simulink model "px4demo_attitude_plant"  (R2017b)
settings: Solver=ode3  StartTime=0.0  StopTime=20  RelTol=1e-3  EnableMultiTasking=on
libraries: aerolibobsolete x1, aerolibatmos2 x1, aerolibnav x1
Description:
  | PX4 PSP Example Model for a Attitude Control/Plant Model
  | 
  | ATTITUDE CONTROL PLANT Top-Level System
settings Model: Creator=skuznick  LastModifiedBy=skuznick
settings DataIOCC: LimitDataPoints=on  SaveFormat=Array
settings OptimizationCC: LifeSpan=1.0
settings DebuggingCC: SolverPrmCheckMsg=warning  AllowSymbolicDim=off  SFUnexpectedBacktrackingDiag=warning  SFNoUnconditionalDefaultTransitionDiag=warning  SFExecutionAtInitializationDiag=none
settings HardwareCC: ProdBitPerPointer=32  ProdBitPerSizeT=32  ProdBitPerPtrDiffT=32  ProdLargestAtomicInteger=Long  ProdLargestAtomicFloat=Double  ProdIntDivRoundTo=Undefined  ProdWordSize=32  ProdHWDeviceType=ARM Compatible->ARM Cortex
settings ModelReferenceCC: PropagateSignalLabelsOutOfModel=off
settings CodeAppCC: StateflowObjectComments=on
settings GRTTargetCC: TargetLangStandard=C89/C90 (ANSI)  GeneratePreprocessorConditionals=Disable all
settings ConfigComp: CovMetricSettings=dw  CovHtmlReporting=on  CovSaveCumulativeToWorkspaceVar=on  CovSaveSingleToWorkspaceVar=on  CovExternalEMLEnable=off  CovSFcnEnable=off

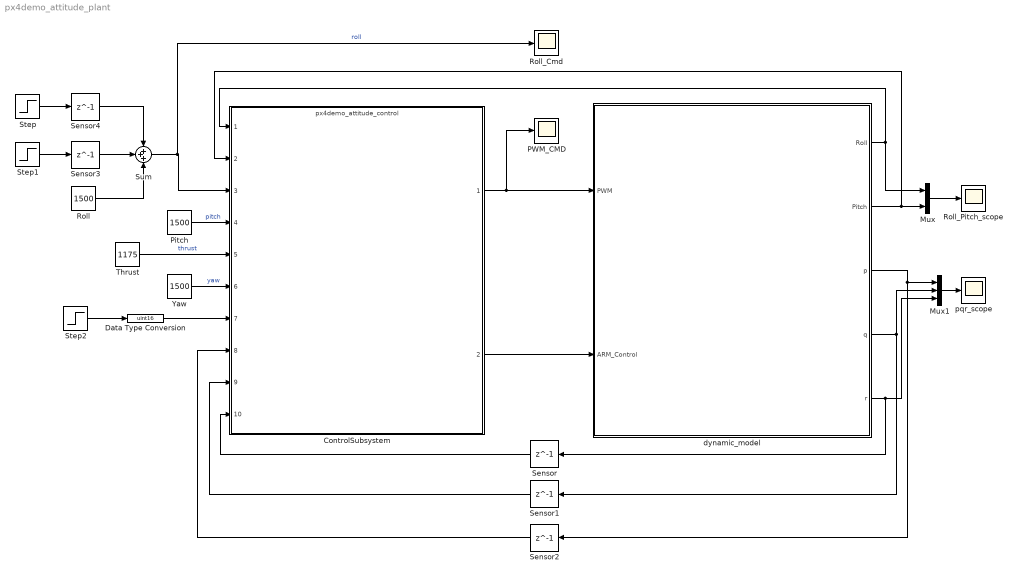
== system px4demo_attitude_plant ==
  ControlSubsystem : ModelReference  ModelNameDialog=px4demo_attitude_control  SimulationMode=Normal  ModelReferenceVersion=1.109
  Data Type Conversion : DataTypeConversion  OutDataTypeStr=uint16
  Mux : Mux  Inputs=2
  Mux1 : Mux  Inputs=3
  PWM_CMD : Scope
  Pitch : Constant  Value=1500  OutDataTypeStr=uint16
  Roll : Constant  Value=1500
  Roll_Cmd : Scope
  Roll_Pitch_scope : Scope
  Sensor{,1..4} (5 alike) : Delay  DelayLength=1
  Step : Step  Time=10  After=100  SampleTime=0
  Step1 : Step  Time=16  After=-100  SampleTime=0
  Step2 : Step  Time=5  Before=1499  After=1501  SampleTime=1/250
  Sum : Sum  Inputs=+++  OutDataTypeStr=uint16
  Thrust : Constant  Value=1175  OutDataTypeStr=uint16
  Yaw : Constant  Value=1500  OutDataTypeStr=uint16
  dynamic_model : Subsystem
  pqr_scope : Scope
  wires:
  dynamic_model/1(Roll) -> ControlSubsystem/1, Mux/1
  dynamic_model/2(Pitch) -> Mux/2, ControlSubsystem/2
  dynamic_model/5(r) -> Mux1/3, Sensor/1
  dynamic_model/4(q) -> Sensor1/1, Mux1/2
  dynamic_model/3(p) -> Mux1/1, Sensor2/1
  Pitch/1 -> ControlSubsystem/4  "pitch"
  Thrust/1 -> ControlSubsystem/5  "thrust"
  Yaw/1 -> ControlSubsystem/6  "yaw"
  Step/1 -> Sensor4/1
  ControlSubsystem/1 -> PWM_CMD/1, dynamic_model/1(PWM)
  Sensor/1 -> ControlSubsystem/10
  Sensor1/1 -> ControlSubsystem/9
  Sensor2/1 -> ControlSubsystem/8
  ControlSubsystem/2 -> dynamic_model/2(ARM_Control)
  Step2/1 -> Data Type Conversion/1
  Sum/1 -> Roll_Cmd/1, ControlSubsystem/3  "roll"
  Sensor4/1 -> Sum/1
  Step1/1 -> Sensor3/1
  Sensor3/1 -> Sum/2
  Roll/1 -> Sum/3
  Mux1/1 -> pqr_scope/1
  Mux/1 -> Roll_Pitch_scope/1
  Data Type Conversion/1 -> ControlSubsystem/7

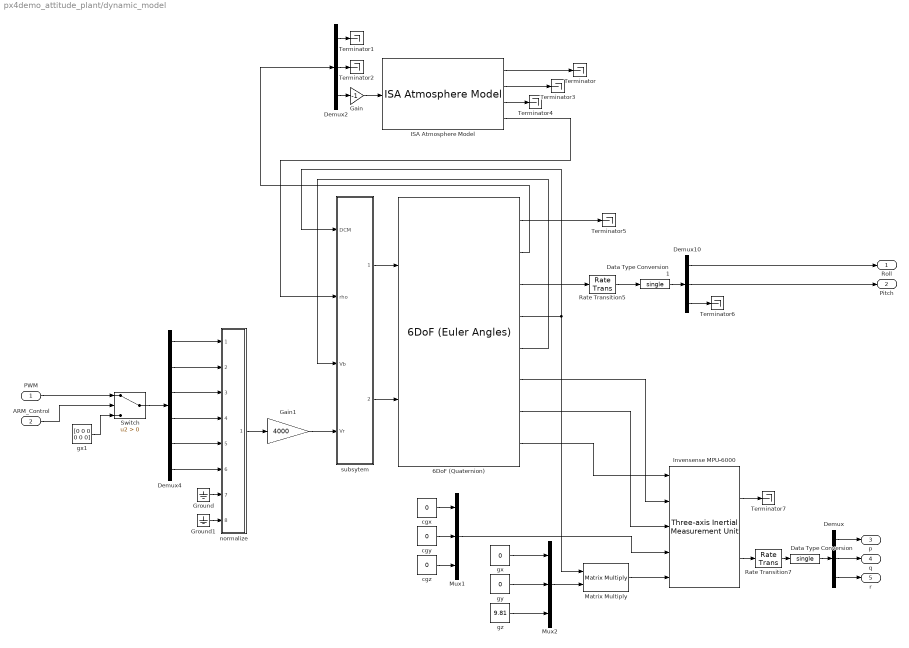
== system px4demo_attitude_plant/dynamic_model ==
  PWM : Inport
  ARM_Control : Inport  Port=2
  6DoF (Quaternion) : aerolibobsolete/6DoF (Euler Angles)  units=Metric (MKS)  mtype=Fixed  rep=Quaternion  xme_0=[0 0 0]  Vm_0=[0 0 0]  eul_0=[0 0 0]  pm_0=[0 0 0]  mass_0=0.26  mass_e=0  mass_f=0  inertia=[0.00080, 0, 0; 0, 0.00065, 0; 0, 0, 0.0014]  inertia_e=eye(3)  inertia_f=eye(3)  k_quat=1.0
      settings: SourceProductName=Aerospace Blockset  SourceProductBaseCode=AE
  Data Type Conversion : DataTypeConversion  OutDataTypeStr=single
  Data Type Conversion1 : DataTypeConversion  OutDataTypeStr=single
  Demux : Demux  Outputs=3
  Demux10 : Demux  Outputs=3
  Demux2 : Demux  Outputs=3
  Demux4 : Demux  Outputs=6
  Gain : Gain  Gain=-1
  Gain1 : Gain  Gain=4000
  Ground : Ground
  Ground1 : Ground
  ISA Atmosphere Model : aerolibatmos2/ISA Atmosphere Model  custom=on  g=9.80665  gamma=1.4  R=287.0531  L=0.0065  h_trop=11000  h_strat=20000  rho0=1.225  P0=101325  T0=288.15  h0=-10
      settings: SourceProductName=Aerospace Blockset
  Invensense MPU-6000 : aerolibnav/Three-axis Inertial Measurement Unit  units=Metric (MKS)  imu=[0 0 0]  dtype_a=off  w_a=190  z_a=0.707  a_sf_cc=[0.98 0 0; 0 0.98 0; 0 0 0.98]  a_bias=[0 0 0]  a_sat="[-19.62  -19.62  -19.62 19.62 19.62 19.62]"  dtype_g=off  w_g=190  z_g=0.707  g_sf_cc=[.98 0 0; 0 .98 0; 0 0 .98]  g_bias=[0 0 0]  g_sens=[0 0 0]  g_sat="[-4.36  -4.36  -4.36 4.36 4.36 4.36]"  i_rand=on  i_seeds=[348631 366719 978432 189621 128794 214632]  i_pow=[0.0000001 0.0000001 0.0000001 0.0000000005 0.0000000005 0.0000000005]  i_Ts=0.004
  Matrix Multiply : Product  Multiplication=Matrix(*)
  Mux1 : Mux  Inputs=3
  Mux2 : Mux  Inputs=3
  Rate Transition5 : RateTransition  OutPortSampleTime=0.004
  Rate Transition7 : RateTransition  OutPortSampleTime=0.004
  Switch : Switch  Criteria=u2 > Threshold
  Terminator{,1..7} (8 alike) : Terminator
      Terminator settings: RequirementInfo="{}  %GIDa_5fc064b5_93ab_4edb_a253_e24b3bd0a00c"
      Terminator3 settings: RequirementInfo="{}  %GIDa_f78a4144_45b0_4cf8_a9c4_4d5b52bd847c"
      Terminator4 settings: RequirementInfo="{}  %GIDa_78a540bb_67c5_46bb_934f_5c1882e1e222"
  cgx : Constant  Value=0
  cgy : Constant  Value=0
  cgz : Constant  Value=0
  gx : Constant  Value=0
  gx1 : Constant  Value=[0 0 0 0 0 0]  OutDataTypeStr=uint16
  gy : Constant  Value=0
  gz : Constant  Value=9.81
  normalize : Subsystem
      mask Display:
      | port_label('input', 1, 'pwm1');
      | port_label('input', 2, 'pwm2');
      | port_label('input', 3, 'pwm3');
      | port_label('input', 4, 'pwm4');
      | port_label('input', 5, 'pwm5');
      | port_label('input', 6, 'pwm6');
      | port_label('input', 7, 'pwm7');
      | port_label('input', 8, 'pwm8');
  subsytem : Subsystem  mask{propD=0.1397, mass=0.26, vehiD=0.25, Cd=0.1}
      mask prompts: propD "Propeller Diameter"; mass "Vehicle Mass"; vehiD "Vehicle Diameter"; Cd "Drag Coefficient"
  Roll : Outport
  Pitch : Outport  Port=2
  p : Outport  Port=3
  q : Outport  Port=4
  r : Outport  Port=5
  wires:
  subsytem/2(moments) -> 6DoF (Quaternion)/2
  subsytem/1(Forces) -> 6DoF (Quaternion)/1
  Invensense MPU-6000/2 -> Rate Transition7/1
  6DoF (Quaternion)/2 -> Demux2/1
  6DoF (Quaternion)/4 -> subsytem/1(DCM), Matrix Multiply/1
  Demux2/1 -> Terminator1/1
  Demux2/2 -> Terminator2/1
  Rate Transition5/1 -> Data Type Conversion1/1
  6DoF (Quaternion)/3 -> Rate Transition5/1
  Demux10/3 -> Terminator6/1
  Demux10/2 -> Pitch/1
  Demux10/1 -> Roll/1
  Gain/1 -> ISA Atmosphere Model/1
  Demux2/3 -> Gain/1
  6DoF (Quaternion)/6 -> Invensense MPU-6000/2
  Demux/3 -> r/1
  Demux/2 -> q/1
  Demux/1 -> p/1
  Mux2/1 -> Matrix Multiply/2
  gz/1 -> Mux2/3
  gx/1 -> Mux2/1
  gy/1 -> Mux2/2
  6DoF (Quaternion)/8 -> Invensense MPU-6000/1
  6DoF (Quaternion)/7 -> Invensense MPU-6000/3
  Mux1/1 -> Invensense MPU-6000/4
  cgz/1 -> Mux1/3
  cgx/1 -> Mux1/1
  cgy/1 -> Mux1/2
  ISA Atmosphere Model/1 -> Terminator/1
  ISA Atmosphere Model/2 -> Terminator3/1
  ISA Atmosphere Model/3 -> Terminator4/1
  6DoF (Quaternion)/1 -> Terminator5/1
  PWM/1 -> Switch/1
  ARM_Control/1 -> Switch/2
  gx1/1 -> Switch/3
  Switch/1 -> Demux4/1
  Invensense MPU-6000/1 -> Terminator7/1
  Demux4/2 -> normalize/2(pwm2)
  Demux4/3 -> normalize/3(pwm3)
  Demux4/6 -> normalize/6(pwm6)
  Demux4/5 -> normalize/5(pwm5)
  Demux4/1 -> normalize/1(pwm1)
  Demux4/4 -> normalize/4(pwm4)
  Ground/1 -> normalize/7(pwm7)
  Ground1/1 -> normalize/8(pwm8)
  normalize/1(normalized_signals) -> Gain1/1
  Gain1/1 -> subsytem/4(Vr)
  Matrix Multiply/1 -> Invensense MPU-6000/5
  6DoF (Quaternion)/5 -> subsytem/3(Vb)
  ISA Atmosphere Model/4 -> subsytem/2(rho)
  Rate Transition7/1 -> Data Type Conversion/1
  Data Type Conversion/1 -> Demux/1
  Data Type Conversion1/1 -> Demux10/1

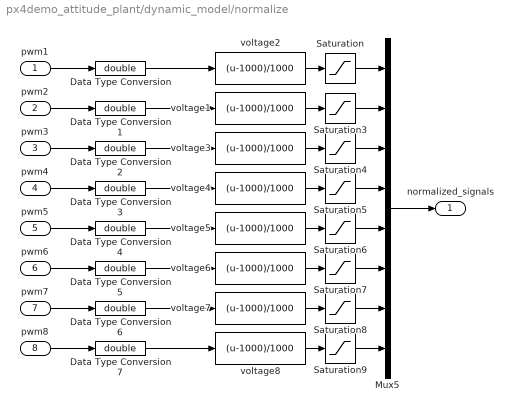
== system px4demo_attitude_plant/dynamic_model/normalize ==
  pwm1 : Inport
  pwm2 : Inport  Port=2
  pwm3 : Inport  Port=3
  pwm4 : Inport  Port=4
  pwm5 : Inport  Port=5
  pwm6 : Inport  Port=6
  pwm7 : Inport  Port=7
  pwm8 : Inport  Port=8
  Data Type Conversion{,1..7} (8 alike) : DataTypeConversion  OutDataTypeStr=double
  Mux5 : Mux  Inputs=8
  Saturation{,3..9} (8 alike) : Saturate  UpperLimit=1  LowerLimit=0
  voltage{1..8} (8 alike) : Fcn  Expr=(u-1000)/1000
  normalized_signals : Outport
  wires:
  voltage1/1 -> Saturation3/1
  Saturation3/1 -> Mux5/2
  Saturation/1 -> Mux5/1
  Saturation6/1 -> Mux5/5
  voltage5/1 -> Saturation6/1
  pwm2/1 -> Data Type Conversion1/1
  pwm5/1 -> Data Type Conversion4/1
  pwm4/1 -> Data Type Conversion3/1
  pwm8/1 -> Data Type Conversion7/1
  pwm6/1 -> Data Type Conversion5/1
  pwm7/1 -> Data Type Conversion6/1
  Saturation4/1 -> Mux5/3
  voltage3/1 -> Saturation4/1
  pwm1/1 -> Data Type Conversion/1
  Mux5/1 -> normalized_signals/1
  pwm3/1 -> Data Type Conversion2/1
  Saturation9/1 -> Mux5/8
  voltage8/1 -> Saturation9/1
  Saturation8/1 -> Mux5/7
  voltage7/1 -> Saturation8/1
  voltage2/1 -> Saturation/1
  voltage4/1 -> Saturation5/1
  voltage6/1 -> Saturation7/1
  Saturation7/1 -> Mux5/6
  Saturation5/1 -> Mux5/4
  Data Type Conversion/1 -> voltage2/1
  Data Type Conversion1/1 -> voltage1/1
  Data Type Conversion2/1 -> voltage3/1
  Data Type Conversion3/1 -> voltage4/1
  Data Type Conversion4/1 -> voltage5/1
  Data Type Conversion5/1 -> voltage6/1
  Data Type Conversion6/1 -> voltage7/1
  Data Type Conversion7/1 -> voltage8/1

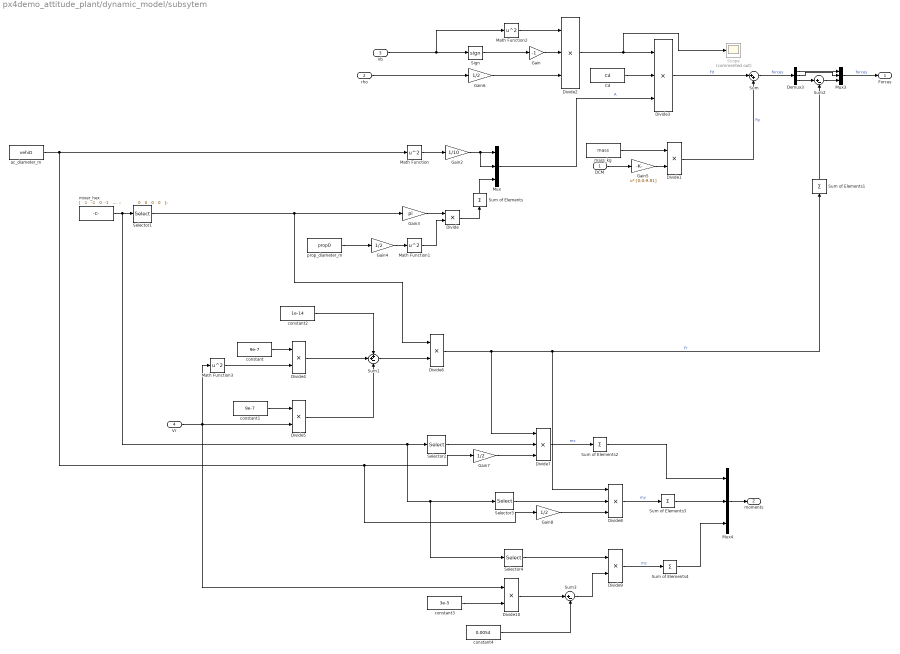
== system px4demo_attitude_plant/dynamic_model/subsytem ==
  DCM : Inport
  rho : Inport  Port=2
  Vb : Inport  Port=3
  Vr : Inport  Port=4
  Cd : Constant  Value=Cd
  Demux3 : Demux  Outputs=3
  Divide{,1,4..6,9..10} (7 alike) : Product  Inputs=**
  Divide{2..3,7..8} (4 alike) : Product  Inputs=***
  Gain : Gain  Gain=-1
  Gain2 : Gain  Gain=1/10
  Gain3 : Gain  Gain=pi
  Gain{4,6..8} (4 alike) : Gain  Gain=1/2
  Gain5 : Gain  Gain=[0;0;9.81]  Multiplication=Matrix(u*K)
  Math Function{,1..3} (4 alike) : Math  Operator=square  SaturateOnIntegerOverflow=on
  Mux : Mux  Inputs=3
  Mux3 : Mux  Inputs=3
  Mux4 : Mux  Inputs=3
  Scope : Scope  Commented=on
  Selector1 : Selector  NumberOfDimensions=2  InputPortWidth=[8 4]  IndexOptions=Index vector (dialog),Index vector (dialog)  Indices=[1:8],1  OutputSizes=1,1
  Selector2 : Selector  NumberOfDimensions=2  InputPortWidth=[8 4]  IndexOptions=Index vector (dialog),Index vector (dialog)  Indices=[1:8],2  OutputSizes=1,1
  Selector3 : Selector  NumberOfDimensions=2  InputPortWidth=[8 4]  IndexOptions=Index vector (dialog),Index vector (dialog)  Indices=[1:8],3  OutputSizes=1,1
  Selector4 : Selector  NumberOfDimensions=2  InputPortWidth=[8 4]  IndexOptions=Index vector (dialog),Index vector (dialog)  Indices=[1:8],4  OutputSizes=1,1
  Sign : Signum
  Sum : Sum  Inputs=|++
  Sum of Elements{,1..4} (5 alike) : Sum  Inputs=+
  Sum1 : Sum  Inputs=++-
  Sum2 : Sum  Inputs=|+-
  Sum3 : Sum  Inputs=|+-
  ac_diameter_m : Constant  Value=vehiD
  constant : Constant  Value=9e-7
  constant1 : Constant  Value=9e-7
  constant2 : Constant  Value=1e-14
  constant3 : Constant  Value=3e-5
  constant4 : Constant  Value=0.0054
  mass_kg : Constant  Value=mass
  mixer_hex : Constant  Value=|
      | [   1   -1   0  -1   ;
      |             1  1   0   1   ;
      |             1  1   1  -1   ;
      |             1  -1  -1   1   ;
      |             1   -1  1  1   ;
      |             1   1   -1   -1   ;
      |             0   0   0   0   ;
      |             0   0   0   0   ];
  prop_diameter_m : Constant  Value=propD
  Forces : Outport
  moments : Outport  Port=2
  wires:
  Math Function/1 -> Gain2/1
  Divide6/1 -> Divide7/1, Divide8/1, Sum of Elements1/1  "Fr"
  Sum/1 -> Demux3/1  "forces"
  constant/1 -> Divide4/1
  constant1/1 -> Divide5/1
  DCM/1 -> Gain5/1
  Divide3/1 -> Sum/1  "Fd"
  mass_kg/1 -> Divide1/1
  Gain5/1 -> Divide1/2
  Sum of Elements/1 -> Mux/3
  Cd/1 -> Divide3/2
  Math Function2/1 -> Divide2/1
  Gain4/1 -> Math Function1/1
  Gain3/1 -> Divide/1
  Divide1/1 -> Sum/2  "Fg"
  Selector1/1 -> Divide6/1, Gain3/1
  Divide/1 -> Sum of Elements/1
  Mux/1 -> Divide3/3  "A"
  prop_diameter_m/1 -> Gain4/1
  Gain6/1 -> Divide2/3
  Math Function1/1 -> Divide/2
  mixer_hex/1 -> Selector4/1, Selector3/1, Selector2/1, Selector1/1
  Gain2/1 -> Mux/2, Mux/1
  ac_diameter_m/1 -> Gain8/1, Gain7/1, Math Function/1
  Selector3/1 -> Divide8/2
  Sum2/1 -> Mux3/3
  Divide4/1 -> Sum1/2
  Vr/1 -> Divide10/1, Math Function3/1, Divide5/2
  Gain7/1 -> Divide7/3
  Sum1/1 -> Divide6/2
  Math Function3/1 -> Divide4/2
  constant2/1 -> Sum1/1
  Divide5/1 -> Sum1/3
  Sum of Elements3/1 -> Mux4/2
  Mux3/1 -> Forces/1  "forces"
  Selector2/1 -> Divide7/2
  Divide10/1 -> Sum3/1
  Demux3/3 -> Sum2/1
  constant4/1 -> Sum3/2
  Divide8/1 -> Sum of Elements3/1  "my"
  Demux3/1 -> Mux3/1
  Sum of Elements2/1 -> Mux4/1
  Selector4/1 -> Divide9/1
  Sum3/1 -> Divide9/2
  Demux3/2 -> Mux3/2
  Sum of Elements1/1 -> Sum2/2
  constant3/1 -> Divide10/2
  Divide7/1 -> Sum of Elements2/1  "mx"
  Gain8/1 -> Divide8/3
  Divide9/1 -> Sum of Elements4/1  "mz"
  Sum of Elements4/1 -> Mux4/3
  Mux4/1 -> moments/1
  Vb/1 -> Sign/1, Math Function2/1
  Divide2/1 -> Scope/1, Divide3/1
  rho/1 -> Gain6/1
  Gain/1 -> Divide2/2
  Sign/1 -> Gain/1
